simulink model "PMSM_Control_Using_FOC_And_SVPWM"  (R2023b)
settings: Solver=ode23t  StartTime=0.0  StopTime=2.5  MaxStep=1e-4  RelTol=1e-3
undefined symbols (not defined in the file): Acid, Ion, Ld, Lead, Lithium, Lq, sigbuilder_block
libraries: slpidlib x58, spsSeriesRLCBranchLib x40, spsVoltageMeasurementLib x34, spsMosfetLib x24, spsBatteryLib x19, spsPWMGeneratorDCDCLib x17, spsCurrentMeasurementLib x15, spsAlphaBetaZerotodq0Lib x14, spsUniversalBridgeLib x14, spsPermanentMagnetSynchronousMachineLib x14, spsSVPWMGenerator2LevelLib x14, spsabctoAlphaBetaZeroLib x14
(part 3 of 3)

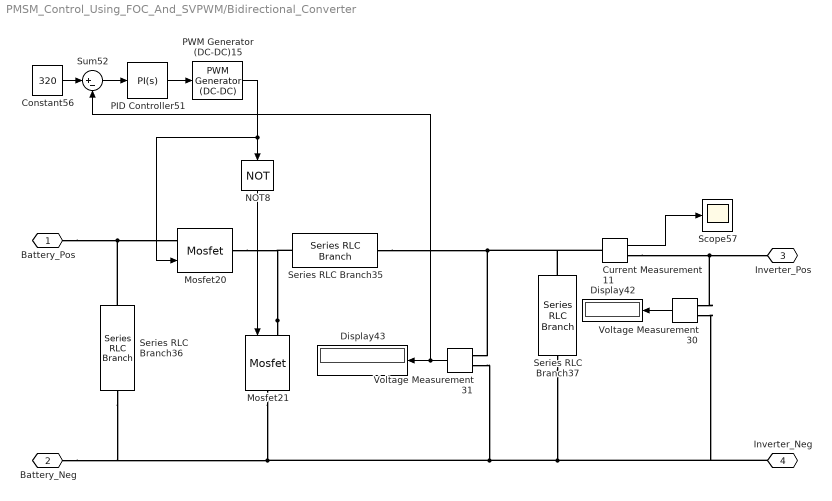
== system PMSM_Control_Using_FOC_And_SVPWM/Bidirectional_Converter ==
  Constant56 : Constant  Value=320
  Current Measurement11 : spsCurrentMeasurementLib/Current Measurement  PhasorSimulation=off  OutputType=Complex  PSBequivalent=0
  Display42 : Display
  Display43 : Display
  Mosfet20 : spsMosfetLib/Mosfet  Ron=0.1  Lon=0  Rd=0.01  Vfd=0  IC=0  Rs=1e5  Cs=inf  Measurements=off
  Mosfet21 : spsMosfetLib/Mosfet  Ron=0.1  Lon=0  Rd=0.01  Vfd=0  IC=0  Rs=1e5  Cs=inf  Measurements=off
  NOT8 : Logic  Operator=NOT  IconShape=distinctive  AllPortsSameDT=off  OutDataTypeStr=boolean
  PID Controller51 : slpidlib/PID Controller  Controller=PI  Form=Parallel  TimeDomain=Continuous-time  UseExternalTs=off  SampleTime=-1  IntegratorMethod=Forward Euler  FilterMethod=Forward Euler  ControllerParametersSource=internal  P=1  I=20  UseKiTs=off  D=0  N=100  UseFilter=on  TunerSelectOption=Transfer Function Based (PID Tuner App)  InitialConditionSource=internal  InitialConditionForIntegrator=0  InitialConditionForFilter=0  DifferentiatorICPrevScaledInput=0  ExternalReset=none  TrackingMode=off  Kt=1  LimitOutput=off  SatLimitsSource=internal  UpperSaturationLimit=inf  LowerSaturationLimit=-inf  LinearizeAsGain=on  AntiWindupMode=none  Kb=1  LimitIntegrator=off  UpperIntegratorSaturationLimit=inf  LowerIntegratorSaturationLimit=-inf  POutMin=[]  POutMax=[]  IOutMin=[]  IOutMax=[]  DOutMin=[]  DOutMax=[]  NOutMin=[]  NOutMax=[]  SumOutMin=[]  SumOutMax=[]  SaturationOutMin=[]  SaturationOutMax=[]  PParamMin=[]  PParamMax=[]  IParamMin=[]  IParamMax=[]  DParamMin=[]  DParamMax=[]  NParamMin=[]  NParamMax=[]  KbParamMin=[]  KbParamMax=[]  KtParamMin=[]  KtParamMax=[]  KbOutMin=[]  KbOutMax=[]  KtOutMin=[]  KtOutMax=[]  IntegratorOutMin=[]  IntegratorOutMax=[]  FilterOutMin=[]  FilterOutMax=[]  SumI1OutMin=[]  SumI1OutMax=[]  SumI2OutMin=[]  SumI2OutMax=[]  SumI3OutMin=[]  SumI3OutMax=[]  SumI4OutMin=[]  SumI4OutMax=[]  SumDOutMin=[]  SumDOutMax=[]  DifferentiatorOutMin=[]  DifferentiatorOutMax=[]  FilterDiffOutCoefMin=[]  FilterDiffOutCoefMax=[]  ReciprocalOutMin=[]  ReciprocalOutMax=[]  SumDenOutMin=[]  SumDenOutMax=[]  SumNumOutMin=[]  SumNumOutMax=[]  DivideOutMin=[]  DivideOutMax=[]  UdiffTsProdOutMin=[]  UdiffTsProdOutMax=[]  NTsProdOutMin=[]  NTsProdOutMax=[]  UintegralTsProdOutMin=[]  UintegralTsProdOutMax=[]  UngainTsProdOutMin=[]  UngainTsProdOutMax=[]  ClampingZeroOutDataTypeStr=Inherit: Inherit via back propagation  ClampingZeroOutMin=[]  ClampingZeroOutMax=[]  FilterDenConstantOutDataTypeStr=Inherit: Inherit via back propagation  FilterDenConstantOutMin=[]  FilterDenConstantOutMax=[]  PCopyOutDataTypeStr=Inherit: Inherit via back propagation  PCopyOutMin=[]  PCopyOutMax=[]  NCopyOutDataTypeStr=Inherit: Inherit via back propagation  NCopyOutMin=[]  NCopyOutMax=[]  IntegratorContinuousStateAttributes=''  IntegratorStateMustResolveToSignalObject=off  IntegratorRTWStateStorageClass=Auto  FilterContinuousStateAttributes=''  FilterStateMustResolveToSignalObject=off  FilterRTWStateStorageClass=Auto  ParallelPVariant=InternalParameters  IdealPVariant=Disabled  IVariant=InternalParameters  DVariant=Disabled  IntegratorVariant=Continuous  SatVariant=Disabled  AWVariant=Passthrough  PCopyVariant=Disabled  TRVariant=Disabled  FdbkBlocksVariant=Forward  IdealPFdbkVariant=Disabled  SatFdbkVariant=Disabled  DerivativeFilterVariant=Disabled  NVariant=Disabled  NCopyVariant=Disabled_SignalSpec  FilterICVariant=Disabled  IntegratorICVariant=InternalICs  ExternalResetVariant=Disabled  TRSumVariant=Passthrough  SumFdbkVariant=Disabled  SumVariant=Sum_PI  TsampFilterVariant=InternalTs  TsampNgainVariant=Passthrough  TsampIntegralVariant=Disabled_SignalSpec  ExternalSaturationOutDataTypeStr=Inherit: Same as second input
  PWM Generator (DC-DC)15 : spsPWMGeneratorDCDCLib/PWM Generator (DC-DC)  Fsw=5000  Ts=0
  Scope57 : Scope
  Series RLC Branch35 : spsSeriesRLCBranchLib/Series RLC Branch  LConnTagsString=__new0  RConnTagsString=__new0  BranchType=L  Resistance=0.0001  Inductance=1e-3  SetiL0=off  InitialCurrent=0  Capacitance=1000e-6  Setx0=off  InitialVoltage=0  Measurements=None
  Series RLC Branch36 : spsSeriesRLCBranchLib/Series RLC Branch  LConnTagsString=__new0  RConnTagsString=__new0  BranchType=RC  Resistance=0.0001  Inductance=1e-3  SetiL0=off  InitialCurrent=0  Capacitance=1000e-6  Setx0=off  InitialVoltage=0  Measurements=None
  Series RLC Branch37 : spsSeriesRLCBranchLib/Series RLC Branch  LConnTagsString=__new0  RConnTagsString=__new0  BranchType=RC  Resistance=0.01  Inductance=1e-3  SetiL0=off  InitialCurrent=0  Capacitance=1e-3  Setx0=off  InitialVoltage=0  Measurements=None
  Sum52 : Sum  Inputs=|+-
  Voltage Measurement30 : spsVoltageMeasurementLib/Voltage Measurement  PhasorSimulation=off  OutputType=Complex  PSBequivalent=0
  Voltage Measurement31 : spsVoltageMeasurementLib/Voltage Measurement  PhasorSimulation=off  OutputType=Complex  PSBequivalent=0
  Battery_Pos : PMIOPort  Side=Left
  Battery_Neg : PMIOPort  Port=2  Side=Left
  Inverter_Pos : PMIOPort  Port=3  Side=Right
  Inverter_Neg : PMIOPort  Port=4  Side=Right
  wires:
  PID Controller51/1 -> PWM Generator (DC-DC)15/1
  Current Measurement11/1 -> Scope57/1
  Constant56/1 -> Sum52/1
  Sum52/1 -> PID Controller51/1
  PWM Generator (DC-DC)15/1 -> Mosfet20/1, NOT8/1
  NOT8/1 -> Mosfet21/1
  Voltage Measurement31/1 -> Sum52/2, Display43/1
  Voltage Measurement30/1 -> Display42/1
  connections:
  Mosfet21/LConn1 -- Series RLC Branch35/LConn1 -- Mosfet20/RConn1
  Series RLC Branch36/LConn1 -- Battery_Pos/RConn1 -- Mosfet20/LConn1
  Current Measurement11/RConn1 -- Voltage Measurement30/LConn1 -- Inverter_Pos/RConn1
  Voltage Measurement31/LConn1 -- Series RLC Branch37/LConn1 -- Current Measurement11/LConn1 -- Series RLC Branch35/RConn1
  Mosfet21/RConn1 -- Voltage Measurement30/LConn2 -- Inverter_Neg/RConn1 -- Series RLC Branch37/RConn1 -- Voltage Measurement31/LConn2 -- Battery_Neg/RConn1 -- Series RLC Branch36/RConn1

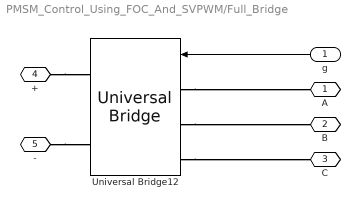
== system PMSM_Control_Using_FOC_And_SVPWM/Full_Bridge ==
  g : Inport
  Universal Bridge12 : spsUniversalBridgeLib/Universal Bridge  Arms=3  SnubberResistance=1e5  SnubberCapacitance=inf  Device=IGBT / Diodes  Ron=1e-3  Lon=0  ForwardVoltages="[  0  0  ]"  ForwardVoltage=0  GTOparameters=[ 10e-6 , 20e-6 ]  IGBTparameters=[ 1e-6 , 2e-6 ]  Measurements=None  Measurements_2=None  converterType=Rectifier
  A : PMIOPort  Side=Left
  B : PMIOPort  Port=2  Side=Left
  C : PMIOPort  Port=3  Side=Left
  + : PMIOPort  Port=4  Side=Right
  - : PMIOPort  Port=5  Side=Right
  wires:
  g/1 -> Universal Bridge12/1
  connections:
  Universal Bridge12/LConn1 -- A/RConn1
  +/RConn1 -- Universal Bridge12/RConn1
  Universal Bridge12/LConn2 -- B/RConn1
  Universal Bridge12/LConn3 -- C/RConn1
  -/RConn1 -- Universal Bridge12/RConn2

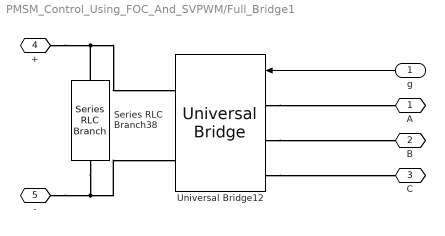
== system PMSM_Control_Using_FOC_And_SVPWM/Full_Bridge1 ==
  g : Inport
  Series RLC Branch38 : spsSeriesRLCBranchLib/Series RLC Branch  LConnTagsString=__new0  RConnTagsString=__new0  BranchType=RC  Resistance=0.01  Inductance=1e-3  SetiL0=off  InitialCurrent=0  Capacitance=1e-3  Setx0=off  InitialVoltage=0  Measurements=None
  Universal Bridge12 : spsUniversalBridgeLib/Universal Bridge  Arms=3  SnubberResistance=1e5  SnubberCapacitance=inf  Device=IGBT / Diodes  Ron=1e-3  Lon=0  ForwardVoltages="[  0  0  ]"  ForwardVoltage=0  GTOparameters=[ 10e-6 , 20e-6 ]  IGBTparameters=[ 1e-6 , 2e-6 ]  Measurements=None  Measurements_2=None  converterType=Rectifier
  A : PMIOPort  Side=Left
  B : PMIOPort  Port=2  Side=Left
  C : PMIOPort  Port=3  Side=Left
  + : PMIOPort  Port=4  Side=Right
  - : PMIOPort  Port=5  Side=Right
  wires:
  g/1 -> Universal Bridge12/1
  connections:
  Universal Bridge12/LConn1 -- A/RConn1
  +/RConn1 -- Series RLC Branch38/LConn1 -- Universal Bridge12/RConn1
  Universal Bridge12/LConn2 -- B/RConn1
  Universal Bridge12/LConn3 -- C/RConn1
  -/RConn1 -- Series RLC Branch38/RConn1 -- Universal Bridge12/RConn2

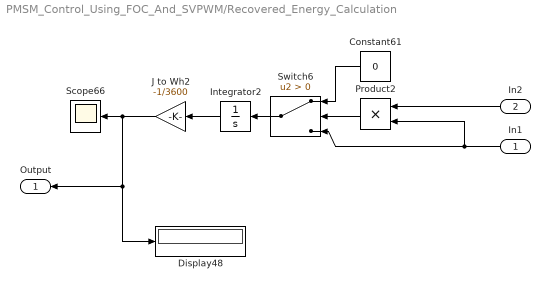
== system PMSM_Control_Using_FOC_And_SVPWM/Recovered_Energy_Calculation ==
  In1 : Inport
  In2 : Inport  Port=2
  Constant61 : Constant  Value=0
  Display48 : Display
  Integrator2 : Integrator
  J to Wh2 : Gain  Gain=-1/3600
  Product2 : Product
  Scope66 : Scope
  Switch6 : Switch  Criteria=u2 > Threshold  SaturateOnIntegerOverflow=off  InputSameDT=off
  Output : Outport
  wires:
  Constant61/1 -> Switch6/1
  Integrator2/1 -> J to Wh2/1
  Switch6/1 -> Integrator2/1
  J to Wh2/1 -> Display48/1, Output/1, Scope66/1
  In2/1 -> Product2/1
  Product2/1 -> Switch6/2
  In1/1 -> Product2/2, Switch6/3

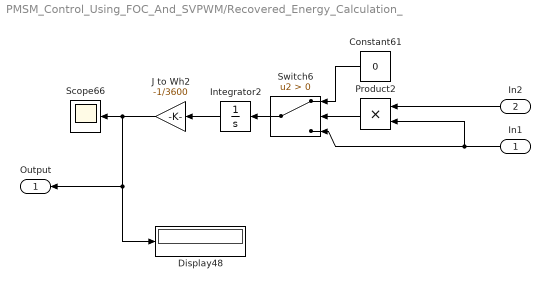
== system PMSM_Control_Using_FOC_And_SVPWM/Recovered_Energy_Calculation_ ==
  In1 : Inport
  In2 : Inport  Port=2
  Constant61 : Constant  Value=0
  Display48 : Display
  Integrator2 : Integrator
  J to Wh2 : Gain  Gain=-1/3600
  Product2 : Product
  Scope66 : Scope
  Switch6 : Switch  Criteria=u2 > Threshold  SaturateOnIntegerOverflow=off  InputSameDT=off
  Output : Outport
  wires:
  Constant61/1 -> Switch6/1
  Integrator2/1 -> J to Wh2/1
  Switch6/1 -> Integrator2/1
  J to Wh2/1 -> Display48/1, Output/1, Scope66/1
  In2/1 -> Product2/1
  Product2/1 -> Switch6/2
  In1/1 -> Product2/2, Switch6/3

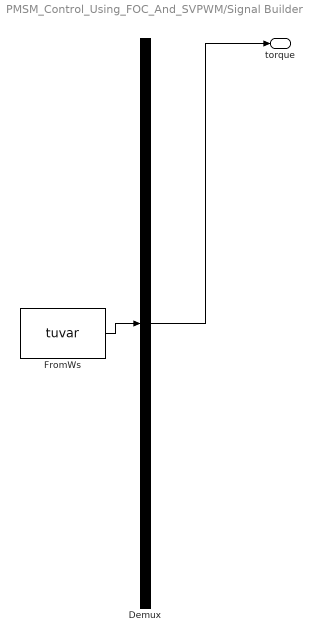
== system PMSM_Control_Using_FOC_And_SVPWM/Signal Builder ==
  Demux : Demux  Tag=STV Demux  Outputs=1
      settings: DisplayOption=none
  FromWs : FromWorkspace  Tag=STV FromWs  VariableName=tuvar
      SigBuilderData=|
      | common.afterFinalStr = 'Extrapolate'
      | common.sampleTime = 0
      | dataSet.timeRange = [0 2.5]
      | dataSet.name = 'Imported_Group 1'
      | sbobj.Name = 'Signal Builder'
      | sbobj.Groups.Name = 'Imported_Group 1'
      | sbobj.Groups.Signals.Name = 'torque'
      | sbobj.Groups.Signals.XData = [0 0.05 0.05 0.5 0.5 0.75 0.75 1.25 1.25 1.65 1.65 2.05 2.05 2.35 2.35 2.5]
      | sbobj.Groups.Signals.YData = [0 0 5 5 4 4 -3 -3 1.5 1.5 5 5 4 4 -1 -1]
      | sbobj.Groups.TimeRange = [0 2.5]
  torque : Outport  VectorParamsAs1DForOutWhenUnconnected=off
  wires:
  Demux/1 -> torque/1
  FromWs/1 -> Demux/1

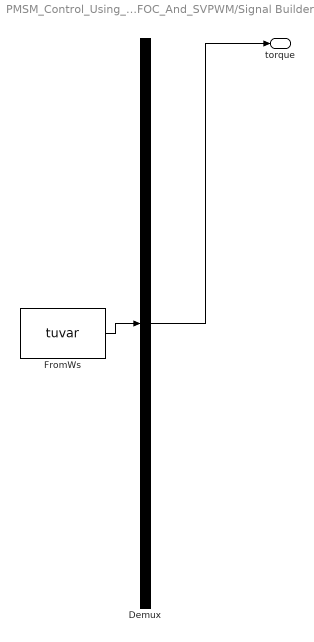
== system PMSM_Control_Using_FOC_And_SVPWM/Signal Builder1 ==
  Demux : Demux  Tag=STV Demux  Outputs=1
      settings: DisplayOption=none
  FromWs : FromWorkspace  Tag=STV FromWs  VariableName=tuvar
      SigBuilderData=|
      | common.afterFinalStr = 'Extrapolate'
      | common.sampleTime = 0
      | dataSet.timeRange = [0 2.5]
      | dataSet.name = 'Imported_Group 1'
      | sbobj.Name = 'Signal Builder'
      | sbobj.Groups.Name = 'Imported_Group 1'
      | sbobj.Groups.Signals.Name = 'torque'
      | sbobj.Groups.Signals.XData = [0 0.05 0.05 0.5 0.5 0.75 0.75 1.25 1.25 1.65 1.65 2.05 2.05 2.35 2.35 2.5]
      | sbobj.Groups.Signals.YData = [0 0 5 5 4 4 -3 -3 1.5 1.5 5 5 4 4 -1 -1]
      | sbobj.Groups.TimeRange = [0 2.5]
  torque : Outport  VectorParamsAs1DForOutWhenUnconnected=off
  wires:
  FromWs/1 -> Demux/1
  Demux/1 -> torque/1

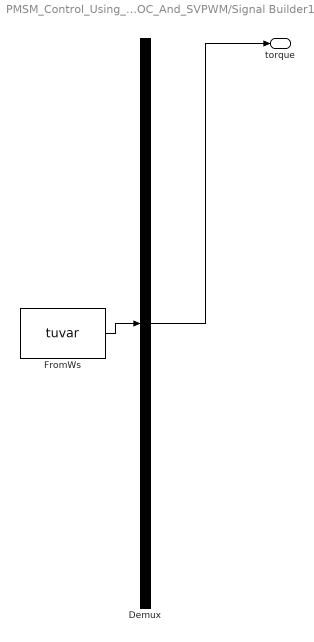
== system PMSM_Control_Using_FOC_And_SVPWM/Signal Builder10 ==
  Demux : Demux  Tag=STV Demux  Outputs=1
      settings: DisplayOption=none
  FromWs : FromWorkspace  Tag=STV FromWs  VariableName=tuvar
      SigBuilderData=|
      | common.afterFinalStr = 'Extrapolate'
      | common.sampleTime = 0
      | dataSet.timeRange = [0 2.5]
      | dataSet.name = 'DownHill_Torque'
      | sbobj.Name = 'Signal Builder'
      | sbobj.Groups.Name = 'DownHill_Torque'
      | sbobj.Groups.Signals.Name = 'torque'
      | sbobj.Groups.Signals.XData = [0 0.05 0.3 0.5 0.8 1.25 1.25 1.65 1.65 2.05 2.35 2.5]
      | sbobj.Groups.Signals.YData = [0 0 -100 -115 -85 -65 -60 -75 -77.5 -50 -40 -1]
      | sbobj.Groups.TimeRange = [0 2.5]
  torque : Outport  VectorParamsAs1DForOutWhenUnconnected=off
  wires:
  FromWs/1 -> Demux/1
  Demux/1 -> torque/1

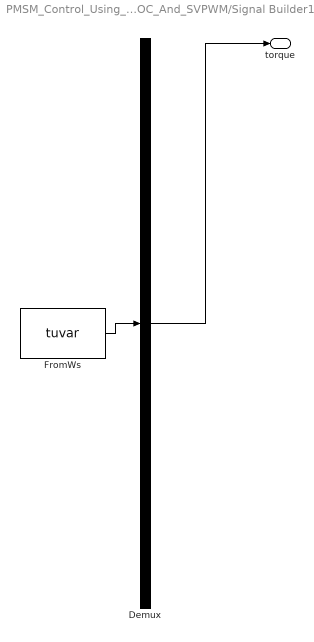
== system PMSM_Control_Using_FOC_And_SVPWM/Signal Builder11 ==
  Demux : Demux  Tag=STV Demux  Outputs=1
      settings: DisplayOption=none
  FromWs : FromWorkspace  Tag=STV FromWs  VariableName=tuvar
      SigBuilderData=|
      | common.afterFinalStr = 'Extrapolate'
      | common.sampleTime = 0
      | dataSet.timeRange = [0 2.5]
      | dataSet.name = 'Flat_Road_Torque'
      | sbobj.Name = 'Signal Builder'
      | sbobj.Groups.Name = 'Flat_Road_Torque'
      | sbobj.Groups.Signals.Name = 'torque'
      | sbobj.Groups.Signals.XData = [0 0.05 0.1 0.3 0.4 0.7 0.8 1.2 1.25 1.6 1.65 2 2.05 2.25 2.35 2.5]
      | sbobj.Groups.Signals.YData = [0 0 8 8 5 5 -8 -8 -3 -3 -7 -7 -8 -8 -1 -1]
      | sbobj.Groups.TimeRange = [0 2.5]
  torque : Outport  VectorParamsAs1DForOutWhenUnconnected=off
  wires:
  FromWs/1 -> Demux/1
  Demux/1 -> torque/1

== system PMSM_Control_Using_FOC_And_SVPWM/Signal Builder13 ==
  Demux : Demux  Tag=STV Demux  Outputs=1
      settings: DisplayOption=none
  FromWs : FromWorkspace  Tag=STV FromWs  VariableName=tuvar
      SigBuilderData=|
      | common.afterFinalStr = 'Extrapolate'
      | common.sampleTime = 0
      | dataSet.timeRange = [0 2.5]
      | dataSet.name = 'Flat_Road_Torque'
      | sbobj.Name = 'Signal Builder'
      | sbobj.Groups.Name = 'Flat_Road_Torque'
      | sbobj.Groups.Signals.Name = 'torque'
      | sbobj.Groups.Signals.XData = [0 0.05 0.1 0.3 0.4 0.7 0.8 1.2 1.25 1.6 1.65 2 2.05 2.25 2.35 2.5]
      | sbobj.Groups.Signals.YData = [0 0 5 5 3 3 -5 -5 -3 -3 -4 -4 -5 -5 -1 -1]
      | sbobj.Groups.TimeRange = [0 2.5]
  torque : Outport  VectorParamsAs1DForOutWhenUnconnected=off
  wires:
  Demux/1 -> torque/1
  FromWs/1 -> Demux/1

== system PMSM_Control_Using_FOC_And_SVPWM/Signal Builder2 ==
  Demux : Demux  Tag=STV Demux  Outputs=1
      settings: DisplayOption=none
  FromWs : FromWorkspace  Tag=STV FromWs  VariableName=tuvar
      SigBuilderData=|
      | common.afterFinalStr = 'Extrapolate'
      | common.sampleTime = 0
      | dataSet.timeRange = [0 2.5]
      | dataSet.name = 'Imported_Group 1'
      | sbobj.Name = 'Signal Builder'
      | sbobj.Groups.Name = 'Imported_Group 1'
      | sbobj.Groups.Signals.Name = 'torque'
      | sbobj.Groups.Signals.XData = [0 0.05 0.05 0.5 0.5 0.75 0.75 1.25 1.25 1.65 1.65 2.05 2.05 2.35 2.35 2.5]
      | sbobj.Groups.Signals.YData = [0 0 5 5 4 4 -3 -3 1.5 1.5 5 5 4 4 -1 -1]
      | sbobj.Groups.TimeRange = [0 2.5]
  torque : Outport  VectorParamsAs1DForOutWhenUnconnected=off
  wires:
  FromWs/1 -> Demux/1
  Demux/1 -> torque/1

== system PMSM_Control_Using_FOC_And_SVPWM/Signal Builder3 ==
  Demux : Demux  Tag=STV Demux  Outputs=1
      settings: DisplayOption=none
  FromWs : FromWorkspace  Tag=STV FromWs  VariableName=tuvar
      SigBuilderData=|
      | common.afterFinalStr = 'Extrapolate'
      | common.sampleTime = 0
      | dataSet.timeRange = [0 2.5]
      | dataSet.name = 'Flat_Road_Torque'
      | sbobj.Name = 'Signal Builder'
      | sbobj.Groups.Name = 'Flat_Road_Torque'
      | sbobj.Groups.Signals.Name = 'torque'
      | sbobj.Groups.Signals.XData = [0 0.05 0.05 0.5 0.5 0.75 0.75 1.25 1.25 1.65 1.65 2.05 2.05 2.35 2.35 2.5]
      | sbobj.Groups.Signals.YData = [0 0 5 5 4 4 -3 -3 1.5 1.5 5 5 4 4 -1 -1]
      | sbobj.Groups.TimeRange = [0 2.5]
  torque : Outport  VectorParamsAs1DForOutWhenUnconnected=off
  wires:
  Demux/1 -> torque/1
  FromWs/1 -> Demux/1

== system PMSM_Control_Using_FOC_And_SVPWM/Signal Builder4 ==
  Demux : Demux  Tag=STV Demux  Outputs=1
      settings: DisplayOption=none
  FromWs : FromWorkspace  Tag=STV FromWs  VariableName=tuvar
      SigBuilderData=|
      | common.afterFinalStr = 'Extrapolate'
      | common.sampleTime = 0
      | dataSet.timeRange = [0 2.5]
      | dataSet.name = 'Imported_Group 1'
      | sbobj.Name = 'Signal Builder'
      | sbobj.Groups.Name = 'Imported_Group 1'
      | sbobj.Groups.Signals.Name = 'torque'
      | sbobj.Groups.Signals.XData = [0 0.05 0.05 0.5 0.5 0.75 0.75 1.25 1.25 1.65 1.65 2.05 2.05 2.35 2.35 2.5]
      | sbobj.Groups.Signals.YData = [0 0 5 5 4 4 -3 -3 1.5 1.5 5 5 4 4 -1 -1]
      | sbobj.Groups.TimeRange = [0 2.5]
  torque : Outport  VectorParamsAs1DForOutWhenUnconnected=off
  wires:
  Demux/1 -> torque/1
  FromWs/1 -> Demux/1

== system PMSM_Control_Using_FOC_And_SVPWM/Signal Builder5 ==
  Demux : Demux  Tag=STV Demux  Outputs=1
      settings: DisplayOption=none
  FromWs : FromWorkspace  Tag=STV FromWs  VariableName=tuvar
      SigBuilderData=|
      | common.afterFinalStr = 'Extrapolate'
      | common.sampleTime = 0
      | dataSet.timeRange = [0 2.5]
      | dataSet.name = 'DownHill_Torque'
      | sbobj.Name = 'Signal Builder'
      | sbobj.Groups.Name = 'DownHill_Torque'
      | sbobj.Groups.Signals.Name = 'torque'
      | sbobj.Groups.Signals.XData = [0 0.05 0.3 0.5 0.8 1.25 1.25 1.65 1.65 2.05 2.35 2.5]
      | sbobj.Groups.Signals.YData = [0 0 -100 -115 -85 -65 -60 -75 -77.5 -50 -40 -1]
      | sbobj.Groups.TimeRange = [0 2.5]
  torque : Outport  VectorParamsAs1DForOutWhenUnconnected=off
  wires:
  Demux/1 -> torque/1
  FromWs/1 -> Demux/1

== system PMSM_Control_Using_FOC_And_SVPWM/Signal Builder6 ==
  Demux : Demux  Tag=STV Demux  Outputs=1
      settings: DisplayOption=none
  FromWs : FromWorkspace  Tag=STV FromWs  VariableName=tuvar
      SigBuilderData=|
      | common.afterFinalStr = 'Extrapolate'
      | common.sampleTime = 0
      | dataSet.timeRange = [0 2.5]
      | dataSet.name = 'Flat_Road_Torque'
      | sbobj.Name = 'Signal Builder'
      | sbobj.Groups.Name = 'Flat_Road_Torque'
      | sbobj.Groups.Signals.Name = 'torque'
      | sbobj.Groups.Signals.XData = [0 0.05 0.05 0.5 0.5 0.75 0.75 1.25 1.25 1.65 1.65 2.05 2.05 2.35 2.35 2.5]
      | sbobj.Groups.Signals.YData = [0 0 5 5 4 4 -3 -3 1.5 1.5 5 5 4 4 -1 -1]
      | sbobj.Groups.TimeRange = [0 2.5]
  torque : Outport  VectorParamsAs1DForOutWhenUnconnected=off
  wires:
  FromWs/1 -> Demux/1
  Demux/1 -> torque/1

== system PMSM_Control_Using_FOC_And_SVPWM/Signal Builder7 ==
  Demux : Demux  Tag=STV Demux  Outputs=1
      settings: DisplayOption=none
  FromWs : FromWorkspace  Tag=STV FromWs  VariableName=tuvar
      SigBuilderData=|
      | common.afterFinalStr = 'Extrapolate'
      | common.sampleTime = 0
      | dataSet.timeRange = [0 2.5]
      | dataSet.name = 'Flat_Road_Torque'
      | sbobj.Name = 'Signal Builder'
      | sbobj.Groups.Name = 'Flat_Road_Torque'
      | sbobj.Groups.Signals.Name = 'torque'
      | sbobj.Groups.Signals.XData = [0 0.05 0.05 0.5 0.5 0.75 0.75 1.25 1.25 1.65 1.65 2.05 2.05 2.35 2.35 2.5]
      | sbobj.Groups.Signals.YData = [0 0 5 5 4 4 -3 -3 1.5 1.5 5 5 4 4 -1 -1]
      | sbobj.Groups.TimeRange = [0 2.5]
  torque : Outport  VectorParamsAs1DForOutWhenUnconnected=off
  wires:
  Demux/1 -> torque/1
  FromWs/1 -> Demux/1

== system PMSM_Control_Using_FOC_And_SVPWM/Signal Builder8 ==
  Demux : Demux  Tag=STV Demux  Outputs=1
      settings: DisplayOption=none
  FromWs : FromWorkspace  Tag=STV FromWs  VariableName=tuvar
      SigBuilderData=|
      | common.afterFinalStr = 'Extrapolate'
      | common.sampleTime = 0
      | dataSet.timeRange = [0 2.5]
      | dataSet.name = 'DownHill_Torque'
      | sbobj.Name = 'Signal Builder'
      | sbobj.Groups.Name = 'DownHill_Torque'
      | sbobj.Groups.Signals.Name = 'torque'
      | sbobj.Groups.Signals.XData = [0 0.05 0.3 0.5 0.8 1.25 1.25 1.65 1.65 2.05 2.35 2.5]
      | sbobj.Groups.Signals.YData = [0 0 -100 -115 -85 -65 -60 -75 -77.5 -50 -40 -1]
      | sbobj.Groups.TimeRange = [0 2.5]
  torque : Outport  VectorParamsAs1DForOutWhenUnconnected=off
  wires:
  Demux/1 -> torque/1
  FromWs/1 -> Demux/1

== system PMSM_Control_Using_FOC_And_SVPWM/Signal Builder9 ==
  Demux : Demux  Tag=STV Demux  Outputs=1
      settings: DisplayOption=none
  FromWs : FromWorkspace  Tag=STV FromWs  VariableName=tuvar
      SigBuilderData=|
      | common.afterFinalStr = 'Extrapolate'
      | common.sampleTime = 0
      | dataSet.timeRange = [0 2.5]
      | dataSet.name = 'UpHill_Torque'
      | sbobj.Name = 'Signal Builder'
      | sbobj.Groups.Name = 'UpHill_Torque'
      | sbobj.Groups.Signals.Name = 'torque'
      | sbobj.Groups.Signals.XData = [0 0.05 0.05 0.2 0.2 0.25 0.25 1.25 1.25 1.65 1.65 2.05 2.05 2.35 2.35 2.5]
      | sbobj.Groups.Signals.YData = [0 0 5 5 4 4 -3 -3 -4.5 -4.5 -5 -5 -4 -4 -1 -1]
      | sbobj.Groups.TimeRange = [0 2.5]
  torque : Outport  VectorParamsAs1DForOutWhenUnconnected=off
  wires:
  Demux/1 -> torque/1
  FromWs/1 -> Demux/1

== system PMSM_Control_Using_FOC_And_SVPWM/Speed_Path ==
  Demux : Demux  Tag=STV Demux  Outputs=1
      settings: DisplayOption=none
  FromWs : FromWorkspace  Tag=STV FromWs  VariableName=tuvar
      SigBuilderData=|
      | common.afterFinalStr = 'Extrapolate'
      | common.sampleTime = 0
      | dataSet.timeRange = [0 2.5]
      | dataSet.name = 'Imported_Group 1'
      | sbobj.Name = 'Signal Builder'
      | sbobj.Groups.Name = 'Imported_Group 1'
      | sbobj.Groups.Signals.Name = 'speed'
      | sbobj.Groups.Signals.XData = [0 0 0.5 0.75 1.25 1.65 2.05 2.35 2.5]
      | sbobj.Groups.Signals.YData = [0 0 2500 2500 1000 1000 2000 2000 1000]
      | sbobj.Groups.TimeRange = [0 2.5]
  speed : Outport  VectorParamsAs1DForOutWhenUnconnected=off
  wires:
  Demux/1 -> speed/1
  FromWs/1 -> Demux/1

== system PMSM_Control_Using_FOC_And_SVPWM/Speed_Path1 ==
  Demux : Demux  Tag=STV Demux  Outputs=1
      settings: DisplayOption=none
  FromWs : FromWorkspace  Tag=STV FromWs  VariableName=tuvar
      SigBuilderData=|
      | common.afterFinalStr = 'Extrapolate'
      | common.sampleTime = 0
      | dataSet.timeRange = [0 2.5]
      | dataSet.name = 'Imported_Group 1'
      | sbobj.Name = 'Signal Builder'
      | sbobj.Groups.Name = 'Imported_Group 1'
      | sbobj.Groups.Signals.Name = 'speed'
      | sbobj.Groups.Signals.XData = [0 0 0.5 0.75 1.25 1.65 2.05 2.35 2.5]
      | sbobj.Groups.Signals.YData = [0 0 2500 2500 1000 1000 2000 2000 1000]
      | sbobj.Groups.TimeRange = [0 2.5]
  speed : Outport  VectorParamsAs1DForOutWhenUnconnected=off
  wires:
  FromWs/1 -> Demux/1
  Demux/1 -> speed/1

== system PMSM_Control_Using_FOC_And_SVPWM/Speed_Path10 ==
  Demux : Demux  Tag=STV Demux  Outputs=1
      settings: DisplayOption=none
  FromWs : FromWorkspace  Tag=STV FromWs  VariableName=tuvar
      SigBuilderData=|
      | common.afterFinalStr = 'Extrapolate'
      | common.sampleTime = 0
      | dataSet.timeRange = [0 2.5]
      | dataSet.name = 'DownHill_Speed'
      | sbobj.Name = 'Signal Builder'
      | sbobj.Groups.Name = 'DownHill_Speed'
      | sbobj.Groups.Signals.Name = 'speed'
      | sbobj.Groups.Signals.XData = [0 0.5 0.75 1.25 1.65 2.05 2.35 2.5]
      | sbobj.Groups.Signals.YData = [0 450 500 350 600 500 300 100]
      | sbobj.Groups.TimeRange = [0 2.5]
  speed : Outport  VectorParamsAs1DForOutWhenUnconnected=off
  wires:
  FromWs/1 -> Demux/1
  Demux/1 -> speed/1

== system PMSM_Control_Using_FOC_And_SVPWM/Speed_Path12 ==
  Demux : Demux  Tag=STV Demux  Outputs=1
      settings: DisplayOption=none
  FromWs : FromWorkspace  Tag=STV FromWs  VariableName=tuvar
      SigBuilderData=|
      | common.afterFinalStr = 'Extrapolate'
      | common.sampleTime = 0
      | dataSet(1).timeRange = [0 2.5]
      | dataSet(1).name = 'Flat_Road_Speed'
      | dataSet(2).timeRange = [0 2.5]
      | dataSet(2).name = 'Flat_Road_Speed1'
      | sbobj.Name = 'Signal Builder'
      | sbobj.Groups(1).Name = 'Flat_Road_Speed'
      | sbobj.Groups(1).Signals.Name = 'speed'
      | sbobj.Groups(1).Signals.XData = [0 0.5 0.75 1 1.3 1.5 2 2.5]
      | sbobj.Groups(1).Signals.YData = [0 1800 1800 1000 1000 1500 1500 0]
      | sbobj.Groups(1).TimeRange = [0 2.5]
      | sbobj.Groups(2).Name = 'Flat_Road_Speed1'
      | sbobj.Groups(2).Signals.Name = 'speed'
      | sbobj.Groups(2).Signals.XData = [0 0.5 0.75 1.25 1.65 2.05 2.35 2.5]
      | sbobj.Groups(2).Signals.YData = [0 2500 2500 1000 1000 2000 2000 1000]
      | sbobj.Groups(2).TimeRange = [0 2.5]
  speed : Outport  VectorParamsAs1DForOutWhenUnconnected=off
  wires:
  Demux/1 -> speed/1
  FromWs/1 -> Demux/1

== system PMSM_Control_Using_FOC_And_SVPWM/Speed_Path2 ==
  Demux : Demux  Tag=STV Demux  Outputs=1
      settings: DisplayOption=none
  FromWs : FromWorkspace  Tag=STV FromWs  VariableName=tuvar
      SigBuilderData=|
      | common.afterFinalStr = 'Extrapolate'
      | common.sampleTime = 0
      | dataSet.timeRange = [0 2.5]
      | dataSet.name = 'Imported_Group 1'
      | sbobj.Name = 'Signal Builder'
      | sbobj.Groups.Name = 'Imported_Group 1'
      | sbobj.Groups.Signals.Name = 'speed'
      | sbobj.Groups.Signals.XData = [0 0.5 0.75 1.25 1.65 2.05 2.35 2.5]
      | sbobj.Groups.Signals.YData = [0 2500 2500 1000 1000 2000 2000 1000]
      | sbobj.Groups.TimeRange = [0 2.5]
  speed : Outport  VectorParamsAs1DForOutWhenUnconnected=off
  wires:
  FromWs/1 -> Demux/1
  Demux/1 -> speed/1

== system PMSM_Control_Using_FOC_And_SVPWM/Speed_Path3 ==
  Demux : Demux  Tag=STV Demux  Outputs=1
      settings: DisplayOption=none
  FromWs : FromWorkspace  Tag=STV FromWs  VariableName=tuvar
      SigBuilderData=|
      | common.afterFinalStr = 'Extrapolate'
      | common.sampleTime = 0
      | dataSet(1).timeRange = [0 2.5]
      | dataSet(1).name = 'Flat_Road_Speed'
      | dataSet(2).timeRange = [0 2.5]
      | dataSet(2).name = 'Flat_Road_Speed1'
      | sbobj.Name = 'Signal Builder'
      | sbobj.Groups(1).Name = 'Flat_Road_Speed'
      | sbobj.Groups(1).Signals.Name = 'speed'
      | sbobj.Groups(1).Signals.XData = [0 0.5 0.75 1 1.5 1.8 2.2 2.5]
      | sbobj.Groups(1).Signals.YData = [0 1200 1200 600 600 1000 1000 200]
      | sbobj.Groups(1).TimeRange = [0 2.5]
      | sbobj.Groups(2).Name = 'Flat_Road_Speed1'
      | sbobj.Groups(2).Signals.Name = 'speed'
      | sbobj.Groups(2).Signals.XData = [0 0.5 0.75 1.25 1.65 2.05 2.35 2.5]
      | sbobj.Groups(2).Signals.YData = [0 2500 2500 1000 1000 2000 2000 1000]
      | sbobj.Groups(2).TimeRange = [0 2.5]
  speed : Outport  VectorParamsAs1DForOutWhenUnconnected=off
  wires:
  FromWs/1 -> Demux/1
  Demux/1 -> speed/1

== system PMSM_Control_Using_FOC_And_SVPWM/Speed_Path4 ==
  Demux : Demux  Tag=STV Demux  Outputs=1
      settings: DisplayOption=none
  FromWs : FromWorkspace  Tag=STV FromWs  VariableName=tuvar
      SigBuilderData=|
      | common.afterFinalStr = 'Extrapolate'
      | common.sampleTime = 0
      | dataSet.timeRange = [0 2.5]
      | dataSet.name = 'Imported_Group 1'
      | sbobj.Name = 'Signal Builder'
      | sbobj.Groups.Name = 'Imported_Group 1'
      | sbobj.Groups.Signals.Name = 'speed'
      | sbobj.Groups.Signals.XData = [0 0.5 0.75 1.25 1.65 2.05 2.35 2.5]
      | sbobj.Groups.Signals.YData = [0 2500 2500 1000 1000 2000 2000 1000]
      | sbobj.Groups.TimeRange = [0 2.5]
  speed : Outport  VectorParamsAs1DForOutWhenUnconnected=off
  wires:
  Demux/1 -> speed/1
  FromWs/1 -> Demux/1

== system PMSM_Control_Using_FOC_And_SVPWM/Speed_Path5 ==
  Demux : Demux  Tag=STV Demux  Outputs=1
      settings: DisplayOption=none
  FromWs : FromWorkspace  Tag=STV FromWs  VariableName=tuvar
      SigBuilderData=|
      | common.afterFinalStr = 'Extrapolate'
      | common.sampleTime = 0
      | dataSet.timeRange = [0 2.5]
      | dataSet.name = 'DownHill_Speed'
      | sbobj.Name = 'Signal Builder'
      | sbobj.Groups.Name = 'DownHill_Speed'
      | sbobj.Groups.Signals.Name = 'speed'
      | sbobj.Groups.Signals.XData = [0 0.5 0.75 1.25 1.65 2.05 2.35 2.5]
      | sbobj.Groups.Signals.YData = [0 450 500 350 600 500 300 100]
      | sbobj.Groups.TimeRange = [0 2.5]
  speed : Outport  VectorParamsAs1DForOutWhenUnconnected=off
  wires:
  Demux/1 -> speed/1
  FromWs/1 -> Demux/1

== system PMSM_Control_Using_FOC_And_SVPWM/Speed_Path6 ==
  Demux : Demux  Tag=STV Demux  Outputs=1
      settings: DisplayOption=none
  FromWs : FromWorkspace  Tag=STV FromWs  VariableName=tuvar
      SigBuilderData=|
      | common.afterFinalStr = 'Extrapolate'
      | common.sampleTime = 0
      | dataSet(1).timeRange = [0 2.5]
      | dataSet(1).name = 'Flat_Road_Speed'
      | dataSet(2).timeRange = [0 2.5]
      | dataSet(2).name = 'Flat_Road_Speed1'
      | sbobj.Name = 'Signal Builder'
      | sbobj.Groups(1).Name = 'Flat_Road_Speed'
      | sbobj.Groups(1).Signals.Name = 'speed'
      | sbobj.Groups(1).Signals.XData = [0 0.5 0.75 1 1.5 1.8 2.2 2.5]
      | sbobj.Groups(1).Signals.YData = [0 1200 1200 600 600 1000 1000 200]
      | sbobj.Groups(1).TimeRange = [0 2.5]
      | sbobj.Groups(2).Name = 'Flat_Road_Speed1'
      | sbobj.Groups(2).Signals.Name = 'speed'
      | sbobj.Groups(2).Signals.XData = [0 0.5 0.75 1.25 1.65 2.05 2.35 2.5]
      | sbobj.Groups(2).Signals.YData = [0 2500 2500 1000 1000 2000 2000 1000]
      | sbobj.Groups(2).TimeRange = [0 2.5]
  speed : Outport  VectorParamsAs1DForOutWhenUnconnected=off
  wires:
  FromWs/1 -> Demux/1
  Demux/1 -> speed/1

== system PMSM_Control_Using_FOC_And_SVPWM/Speed_Path7 ==
  Demux : Demux  Tag=STV Demux  Outputs=1
      settings: DisplayOption=none
  FromWs : FromWorkspace  Tag=STV FromWs  VariableName=tuvar
      SigBuilderData=|
      | common.afterFinalStr = 'Extrapolate'
      | common.sampleTime = 0
      | dataSet(1).timeRange = [0 2.5]
      | dataSet(1).name = 'Flat_Road_Speed'
      | dataSet(2).timeRange = [0 2.5]
      | dataSet(2).name = 'Flat_Road_Speed1'
      | sbobj.Name = 'Signal Builder'
      | sbobj.Groups(1).Name = 'Flat_Road_Speed'
      | sbobj.Groups(1).Signals.Name = 'speed'
      | sbobj.Groups(1).Signals.XData = [0 0.5 0.75 1 1.5 1.8 2.2 2.5]
      | sbobj.Groups(1).Signals.YData = [0 1200 1200 600 600 1000 1000 200]
      | sbobj.Groups(1).TimeRange = [0 2.5]
      | sbobj.Groups(2).Name = 'Flat_Road_Speed1'
      | sbobj.Groups(2).Signals.Name = 'speed'
      | sbobj.Groups(2).Signals.XData = [0 0.5 0.75 1.25 1.65 2.05 2.35 2.5]
      | sbobj.Groups(2).Signals.YData = [0 2500 2500 1000 1000 2000 2000 1000]
      | sbobj.Groups(2).TimeRange = [0 2.5]
  speed : Outport  VectorParamsAs1DForOutWhenUnconnected=off
  wires:
  Demux/1 -> speed/1
  FromWs/1 -> Demux/1

== system PMSM_Control_Using_FOC_And_SVPWM/Speed_Path8 ==
  Demux : Demux  Tag=STV Demux  Outputs=1
      settings: DisplayOption=none
  FromWs : FromWorkspace  Tag=STV FromWs  VariableName=tuvar
      SigBuilderData=|
      | common.afterFinalStr = 'Extrapolate'
      | common.sampleTime = 0
      | dataSet.timeRange = [0 2.5]
      | dataSet.name = 'DownHill_Speed'
      | sbobj.Name = 'Signal Builder'
      | sbobj.Groups.Name = 'DownHill_Speed'
      | sbobj.Groups.Signals.Name = 'speed'
      | sbobj.Groups.Signals.XData = [0 0.5 0.75 1.25 1.65 2.05 2.35 2.5]
      | sbobj.Groups.Signals.YData = [0 450 500 350 600 500 300 100]
      | sbobj.Groups.TimeRange = [0 2.5]
  speed : Outport  VectorParamsAs1DForOutWhenUnconnected=off
  wires:
  Demux/1 -> speed/1
  FromWs/1 -> Demux/1

== system PMSM_Control_Using_FOC_And_SVPWM/Speed_Path9 ==
  Demux : Demux  Tag=STV Demux  Outputs=1
      settings: DisplayOption=none
  FromWs : FromWorkspace  Tag=STV FromWs  VariableName=tuvar
      SigBuilderData=|
      | common.afterFinalStr = 'Extrapolate'
      | common.sampleTime = 0
      | dataSet.timeRange = [0 2.5]
      | dataSet.name = 'UpHill_Speed'
      | sbobj.Name = 'Signal Builder'
      | sbobj.Groups.Name = 'UpHill_Speed'
      | sbobj.Groups.Signals.Name = 'speed'
      | sbobj.Groups.Signals.XData = [0 0.5 0.75 1.25 1.65 2.05 2.35 2.5]
      | sbobj.Groups.Signals.YData = [0 2500 2500 1400 1400 800 600 100]
      | sbobj.Groups.TimeRange = [0 2.5]
  speed : Outport  VectorParamsAs1DForOutWhenUnconnected=off
  wires:
  Demux/1 -> speed/1
  FromWs/1 -> Demux/1

== system PMSM_Control_Using_FOC_And_SVPWM/Speed_Ref ==
  Demux : Demux  Tag=STV Demux  Outputs=1
      settings: DisplayOption=none
  FromWs : FromWorkspace  Tag=STV FromWs  VariableName=tuvar
      SigBuilderData=|
      | common.afterFinalStr = 'Extrapolate'
      | common.sampleTime = 0
      | dataSet(1).timeRange = [0 2.5]
      | dataSet(1).name = 'Flat_Road_Speed'
      | dataSet(2).timeRange = [0 2.5]
      | dataSet(2).name = 'Flat_Road_Speed1'
      | sbobj.Name = 'Signal Builder'
      | sbobj.Groups(1).Name = 'Flat_Road_Speed'
      | sbobj.Groups(1).Signals.Name = 'speed'
      | sbobj.Groups(1).Signals.XData = [0 0.5 0.75 1 1.3 1.5 2 2.5]
      | sbobj.Groups(1).Signals.YData = [0 1800 1800 1000 1000 1500 1500 0]
      | sbobj.Groups(1).TimeRange = [0 2.5]
      | sbobj.Groups(2).Name = 'Flat_Road_Speed1'
      | sbobj.Groups(2).Signals.Name = 'speed'
      | sbobj.Groups(2).Signals.XData = [0 0.5 0.75 1.25 1.65 2.05 2.35 2.5]
      | sbobj.Groups(2).Signals.YData = [0 2500 2500 1000 1000 2000 2000 1000]
      | sbobj.Groups(2).TimeRange = [0 2.5]
  speed : Outport  VectorParamsAs1DForOutWhenUnconnected=off
  wires:
  FromWs/1 -> Demux/1
  Demux/1 -> speed/1

== system PMSM_Control_Using_FOC_And_SVPWM/Speed_Ref1 ==
  Demux : Demux  Tag=STV Demux  Outputs=1
      settings: DisplayOption=none
  FromWs : FromWorkspace  Tag=STV FromWs  VariableName=tuvar
      SigBuilderData=|
      | common.afterFinalStr = 'Extrapolate'
      | common.sampleTime = 0
      | dataSet(1).timeRange = [0 2.5]
      | dataSet(1).name = 'Flat_Road_Speed'
      | dataSet(2).timeRange = [0 2.5]
      | dataSet(2).name = 'Flat_Road_Speed1'
      | sbobj.Name = 'Signal Builder'
      | sbobj.Groups(1).Name = 'Flat_Road_Speed'
      | sbobj.Groups(1).Signals.Name = 'speed'
      | sbobj.Groups(1).Signals.XData = [0 0.5 0.75 1 1.3 1.5 2 2.5]
      | sbobj.Groups(1).Signals.YData = [0 1800 1800 1000 1000 1500 1500 0]
      | sbobj.Groups(1).TimeRange = [0 2.5]
      | sbobj.Groups(2).Name = 'Flat_Road_Speed1'
      | sbobj.Groups(2).Signals.Name = 'speed'
      | sbobj.Groups(2).Signals.XData = [0 0.5 0.75 1.25 1.65 2.05 2.35 2.5]
      | sbobj.Groups(2).Signals.YData = [0 2500 2500 1000 1000 2000 2000 1000]
      | sbobj.Groups(2).TimeRange = [0 2.5]
  speed : Outport  VectorParamsAs1DForOutWhenUnconnected=off
  wires:
  FromWs/1 -> Demux/1
  Demux/1 -> speed/1

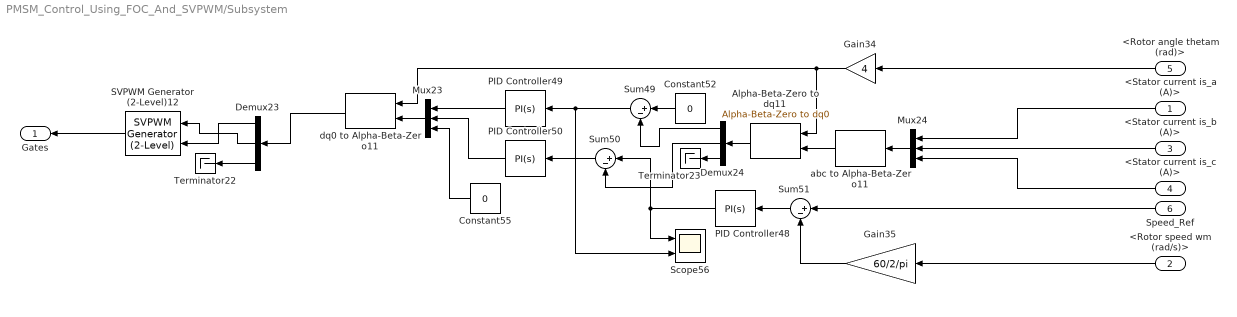
== system PMSM_Control_Using_FOC_And_SVPWM/Subsystem ==
  <Stator current is_a (A)> : Inport
  <Rotor speed wm (rad/s)> : Inport  Port=2
  <Stator current is_b (A)> : Inport  Port=3
  <Stator current is_c (A)> : Inport  Port=4
  <Rotor angle thetam (rad)> : Inport  Port=5
  Speed_Ref : Inport  Port=6
  Alpha-Beta-Zero to dq11 : spsAlphaBetaZerotodq0Lib/Alpha-Beta-Zero to dq0  Alignment=90 degrees behind phase A axis
  Constant52 : Constant  Value=0
  Constant55 : Constant  Value=0
  Demux23 : Demux  Outputs=3
  Demux24 : Demux  Outputs=3
  Gain34 : Gain  Gain=4
  Gain35 : Gain  Gain=60/2/pi
  Mux23 : Mux  Inputs=3
  Mux24 : Mux  Inputs=3
  PID Controller48 : slpidlib/PID Controller  Controller=PI  Form=Parallel  TimeDomain=Continuous-time  UseExternalTs=off  SampleTime=-1  IntegratorMethod=Forward Euler  FilterMethod=Forward Euler  ControllerParametersSource=internal  P=0.5  I=10  UseKiTs=off  D=0  N=100  UseFilter=on  TunerSelectOption=Transfer Function Based (PID Tuner App)  InitialConditionSource=internal  InitialConditionForIntegrator=0  InitialConditionForFilter=0  DifferentiatorICPrevScaledInput=0  ExternalReset=none  TrackingMode=off  Kt=1  LimitOutput=off  SatLimitsSource=internal  UpperSaturationLimit=inf  LowerSaturationLimit=-inf  LinearizeAsGain=on  AntiWindupMode=none  Kb=1  LimitIntegrator=off  UpperIntegratorSaturationLimit=inf  LowerIntegratorSaturationLimit=-inf  POutMin=[]  POutMax=[]  IOutMin=[]  IOutMax=[]  DOutMin=[]  DOutMax=[]  NOutMin=[]  NOutMax=[]  SumOutMin=[]  SumOutMax=[]  SaturationOutMin=[]  SaturationOutMax=[]  PParamMin=[]  PParamMax=[]  IParamMin=[]  IParamMax=[]  DParamMin=[]  DParamMax=[]  NParamMin=[]  NParamMax=[]  KbParamMin=[]  KbParamMax=[]  KtParamMin=[]  KtParamMax=[]  KbOutMin=[]  KbOutMax=[]  KtOutMin=[]  KtOutMax=[]  IntegratorOutMin=[]  IntegratorOutMax=[]  FilterOutMin=[]  FilterOutMax=[]  SumI1OutMin=[]  SumI1OutMax=[]  SumI2OutMin=[]  SumI2OutMax=[]  SumI3OutMin=[]  SumI3OutMax=[]  SumI4OutMin=[]  SumI4OutMax=[]  SumDOutMin=[]  SumDOutMax=[]  DifferentiatorOutMin=[]  DifferentiatorOutMax=[]  FilterDiffOutCoefMin=[]  FilterDiffOutCoefMax=[]  ReciprocalOutMin=[]  ReciprocalOutMax=[]  SumDenOutMin=[]  SumDenOutMax=[]  SumNumOutMin=[]  SumNumOutMax=[]  DivideOutMin=[]  DivideOutMax=[]  UdiffTsProdOutMin=[]  UdiffTsProdOutMax=[]  NTsProdOutMin=[]  NTsProdOutMax=[]  UintegralTsProdOutMin=[]  UintegralTsProdOutMax=[]  UngainTsProdOutMin=[]  UngainTsProdOutMax=[]  ClampingZeroOutDataTypeStr=Inherit: Inherit via back propagation  ClampingZeroOutMin=[]  ClampingZeroOutMax=[]  FilterDenConstantOutDataTypeStr=Inherit: Inherit via back propagation  FilterDenConstantOutMin=[]  FilterDenConstantOutMax=[]  PCopyOutDataTypeStr=Inherit: Inherit via back propagation  PCopyOutMin=[]  PCopyOutMax=[]  NCopyOutDataTypeStr=Inherit: Inherit via back propagation  NCopyOutMin=[]  NCopyOutMax=[]  IntegratorContinuousStateAttributes=''  IntegratorStateMustResolveToSignalObject=off  IntegratorRTWStateStorageClass=Auto  FilterContinuousStateAttributes=''  FilterStateMustResolveToSignalObject=off  FilterRTWStateStorageClass=Auto  ParallelPVariant=InternalParameters  IdealPVariant=Disabled  IVariant=InternalParameters  DVariant=Disabled  IntegratorVariant=Continuous  SatVariant=Disabled  AWVariant=Passthrough  PCopyVariant=Disabled  TRVariant=Disabled  FdbkBlocksVariant=Forward  IdealPFdbkVariant=Disabled  SatFdbkVariant=Disabled  DerivativeFilterVariant=Disabled  NVariant=Disabled  NCopyVariant=Disabled_SignalSpec  FilterICVariant=Disabled  IntegratorICVariant=InternalICs  ExternalResetVariant=Disabled  TRSumVariant=Passthrough  SumFdbkVariant=Disabled  SumVariant=Sum_PI  TsampFilterVariant=InternalTs  TsampNgainVariant=Passthrough  TsampIntegralVariant=Disabled_SignalSpec  ExternalSaturationOutDataTypeStr=Inherit: Same as second input
  PID Controller49 : slpidlib/PID Controller  Controller=PI  Form=Parallel  TimeDomain=Continuous-time  UseExternalTs=off  SampleTime=-1  IntegratorMethod=Forward Euler  FilterMethod=Forward Euler  ControllerParametersSource=internal  P=10  I=2000  UseKiTs=off  D=0  N=100  UseFilter=on  TunerSelectOption=Transfer Function Based (PID Tuner App)  InitialConditionSource=internal  InitialConditionForIntegrator=0  InitialConditionForFilter=0  DifferentiatorICPrevScaledInput=0  ExternalReset=none  TrackingMode=off  Kt=1  LimitOutput=off  SatLimitsSource=internal  UpperSaturationLimit=inf  LowerSaturationLimit=-inf  LinearizeAsGain=on  AntiWindupMode=none  Kb=1  LimitIntegrator=off  UpperIntegratorSaturationLimit=inf  LowerIntegratorSaturationLimit=-inf  POutMin=[]  POutMax=[]  IOutMin=[]  IOutMax=[]  DOutMin=[]  DOutMax=[]  NOutMin=[]  NOutMax=[]  SumOutMin=[]  SumOutMax=[]  SaturationOutMin=[]  SaturationOutMax=[]  PParamMin=[]  PParamMax=[]  IParamMin=[]  IParamMax=[]  DParamMin=[]  DParamMax=[]  NParamMin=[]  NParamMax=[]  KbParamMin=[]  KbParamMax=[]  KtParamMin=[]  KtParamMax=[]  KbOutMin=[]  KbOutMax=[]  KtOutMin=[]  KtOutMax=[]  IntegratorOutMin=[]  IntegratorOutMax=[]  FilterOutMin=[]  FilterOutMax=[]  SumI1OutMin=[]  SumI1OutMax=[]  SumI2OutMin=[]  SumI2OutMax=[]  SumI3OutMin=[]  SumI3OutMax=[]  SumI4OutMin=[]  SumI4OutMax=[]  SumDOutMin=[]  SumDOutMax=[]  DifferentiatorOutMin=[]  DifferentiatorOutMax=[]  FilterDiffOutCoefMin=[]  FilterDiffOutCoefMax=[]  ReciprocalOutMin=[]  ReciprocalOutMax=[]  SumDenOutMin=[]  SumDenOutMax=[]  SumNumOutMin=[]  SumNumOutMax=[]  DivideOutMin=[]  DivideOutMax=[]  UdiffTsProdOutMin=[]  UdiffTsProdOutMax=[]  NTsProdOutMin=[]  NTsProdOutMax=[]  UintegralTsProdOutMin=[]  UintegralTsProdOutMax=[]  UngainTsProdOutMin=[]  UngainTsProdOutMax=[]  ClampingZeroOutDataTypeStr=Inherit: Inherit via back propagation  ClampingZeroOutMin=[]  ClampingZeroOutMax=[]  FilterDenConstantOutDataTypeStr=Inherit: Inherit via back propagation  FilterDenConstantOutMin=[]  FilterDenConstantOutMax=[]  PCopyOutDataTypeStr=Inherit: Inherit via back propagation  PCopyOutMin=[]  PCopyOutMax=[]  NCopyOutDataTypeStr=Inherit: Inherit via back propagation  NCopyOutMin=[]  NCopyOutMax=[]  IntegratorContinuousStateAttributes=''  IntegratorStateMustResolveToSignalObject=off  IntegratorRTWStateStorageClass=Auto  FilterContinuousStateAttributes=''  FilterStateMustResolveToSignalObject=off  FilterRTWStateStorageClass=Auto  ParallelPVariant=InternalParameters  IdealPVariant=Disabled  IVariant=InternalParameters  DVariant=Disabled  IntegratorVariant=Continuous  SatVariant=Disabled  AWVariant=Passthrough  PCopyVariant=Disabled  TRVariant=Disabled  FdbkBlocksVariant=Forward  IdealPFdbkVariant=Disabled  SatFdbkVariant=Disabled  DerivativeFilterVariant=Disabled  NVariant=Disabled  NCopyVariant=Disabled_SignalSpec  FilterICVariant=Disabled  IntegratorICVariant=InternalICs  ExternalResetVariant=Disabled  TRSumVariant=Passthrough  SumFdbkVariant=Disabled  SumVariant=Sum_PI  TsampFilterVariant=InternalTs  TsampNgainVariant=Passthrough  TsampIntegralVariant=Disabled_SignalSpec  ExternalSaturationOutDataTypeStr=Inherit: Same as second input
  PID Controller50 : slpidlib/PID Controller  Controller=PI  Form=Parallel  TimeDomain=Continuous-time  UseExternalTs=off  SampleTime=-1  IntegratorMethod=Forward Euler  FilterMethod=Forward Euler  ControllerParametersSource=internal  P=10  I=2000  UseKiTs=off  D=0  N=100  UseFilter=on  TunerSelectOption=Transfer Function Based (PID Tuner App)  InitialConditionSource=internal  InitialConditionForIntegrator=0  InitialConditionForFilter=0  DifferentiatorICPrevScaledInput=0  ExternalReset=none  TrackingMode=off  Kt=1  LimitOutput=off  SatLimitsSource=internal  UpperSaturationLimit=inf  LowerSaturationLimit=-inf  LinearizeAsGain=on  AntiWindupMode=none  Kb=1  LimitIntegrator=off  UpperIntegratorSaturationLimit=inf  LowerIntegratorSaturationLimit=-inf  POutMin=[]  POutMax=[]  IOutMin=[]  IOutMax=[]  DOutMin=[]  DOutMax=[]  NOutMin=[]  NOutMax=[]  SumOutMin=[]  SumOutMax=[]  SaturationOutMin=[]  SaturationOutMax=[]  PParamMin=[]  PParamMax=[]  IParamMin=[]  IParamMax=[]  DParamMin=[]  DParamMax=[]  NParamMin=[]  NParamMax=[]  KbParamMin=[]  KbParamMax=[]  KtParamMin=[]  KtParamMax=[]  KbOutMin=[]  KbOutMax=[]  KtOutMin=[]  KtOutMax=[]  IntegratorOutMin=[]  IntegratorOutMax=[]  FilterOutMin=[]  FilterOutMax=[]  SumI1OutMin=[]  SumI1OutMax=[]  SumI2OutMin=[]  SumI2OutMax=[]  SumI3OutMin=[]  SumI3OutMax=[]  SumI4OutMin=[]  SumI4OutMax=[]  SumDOutMin=[]  SumDOutMax=[]  DifferentiatorOutMin=[]  DifferentiatorOutMax=[]  FilterDiffOutCoefMin=[]  FilterDiffOutCoefMax=[]  ReciprocalOutMin=[]  ReciprocalOutMax=[]  SumDenOutMin=[]  SumDenOutMax=[]  SumNumOutMin=[]  SumNumOutMax=[]  DivideOutMin=[]  DivideOutMax=[]  UdiffTsProdOutMin=[]  UdiffTsProdOutMax=[]  NTsProdOutMin=[]  NTsProdOutMax=[]  UintegralTsProdOutMin=[]  UintegralTsProdOutMax=[]  UngainTsProdOutMin=[]  UngainTsProdOutMax=[]  ClampingZeroOutDataTypeStr=Inherit: Inherit via back propagation  ClampingZeroOutMin=[]  ClampingZeroOutMax=[]  FilterDenConstantOutDataTypeStr=Inherit: Inherit via back propagation  FilterDenConstantOutMin=[]  FilterDenConstantOutMax=[]  PCopyOutDataTypeStr=Inherit: Inherit via back propagation  PCopyOutMin=[]  PCopyOutMax=[]  NCopyOutDataTypeStr=Inherit: Inherit via back propagation  NCopyOutMin=[]  NCopyOutMax=[]  IntegratorContinuousStateAttributes=''  IntegratorStateMustResolveToSignalObject=off  IntegratorRTWStateStorageClass=Auto  FilterContinuousStateAttributes=''  FilterStateMustResolveToSignalObject=off  FilterRTWStateStorageClass=Auto  ParallelPVariant=InternalParameters  IdealPVariant=Disabled  IVariant=InternalParameters  DVariant=Disabled  IntegratorVariant=Continuous  SatVariant=Disabled  AWVariant=Passthrough  PCopyVariant=Disabled  TRVariant=Disabled  FdbkBlocksVariant=Forward  IdealPFdbkVariant=Disabled  SatFdbkVariant=Disabled  DerivativeFilterVariant=Disabled  NVariant=Disabled  NCopyVariant=Disabled_SignalSpec  FilterICVariant=Disabled  IntegratorICVariant=InternalICs  ExternalResetVariant=Disabled  TRSumVariant=Passthrough  SumFdbkVariant=Disabled  SumVariant=Sum_PI  TsampFilterVariant=InternalTs  TsampNgainVariant=Passthrough  TsampIntegralVariant=Disabled_SignalSpec  ExternalSaturationOutDataTypeStr=Inherit: Same as second input
  SVPWM Generator (2-Level)12 : spsSVPWMGenerator2LevelLib/SVPWM Generator (2-Level)  InputType=alpha-beta components  SwitchingPattern=Pattern #1  Fc=5000  ParUref=[0.8 -30 50]  Ts=0
  Scope56 : Scope  NumInputPorts=2
  Sum49 : Sum  Inputs=|+-
  Sum50 : Sum  Inputs=|+-
  Sum51 : Sum  Inputs=|+-
  Terminator22 : Terminator
  Terminator23 : Terminator
  abc to Alpha-Beta-Zero11 : spsabctoAlphaBetaZeroLib/abc to Alpha-Beta-Zero
  dq0 to Alpha-Beta-Zero11 : spsdq0toAlphaBetaZeroLib/dq0 to Alpha-Beta-Zero  Alignment=90 degrees behind phase A axis
  Gates : Outport
  wires:
  <Rotor angle thetam (rad)>/1 -> Gain34/1
  Mux23/1 -> dq0 to Alpha-Beta-Zero11/1
  Demux24/3 -> Terminator23/1
  Alpha-Beta-Zero to dq11/1 -> Demux24/1
  Constant55/1 -> Mux23/3
  Demux24/2 -> Sum50/2
  Mux24/1 -> abc to Alpha-Beta-Zero11/1
  <Rotor speed wm (rad/s)>/1 -> Gain35/1
  Constant52/1 -> Sum49/1
  Sum51/1 -> PID Controller48/1
  Gain34/1 -> Alpha-Beta-Zero to dq11/2, dq0 to Alpha-Beta-Zero11/2
  Gain35/1 -> Sum51/2
  PID Controller49/1 -> Mux23/1
  SVPWM Generator (2-Level)12/1 -> Gates/1
  abc to Alpha-Beta-Zero11/1 -> Alpha-Beta-Zero to dq11/1
  <Stator current is_a (A)>/1 -> Mux24/1
  <Stator current is_c (A)>/1 -> Mux24/3
  PID Controller50/1 -> Mux23/2
  dq0 to Alpha-Beta-Zero11/1 -> Demux23/1
  <Stator current is_b (A)>/1 -> Mux24/2
  Demux23/1 -> SVPWM Generator (2-Level)12/1
  Sum49/1 -> Scope56/2, PID Controller49/1
  Demux24/1 -> Sum49/2
  Demux23/2 -> SVPWM Generator (2-Level)12/2
  Speed_Ref/1 -> Sum51/1
  Demux23/3 -> Terminator22/1
  Sum50/1 -> PID Controller50/1
  PID Controller48/1 -> Scope56/1, Sum50/1

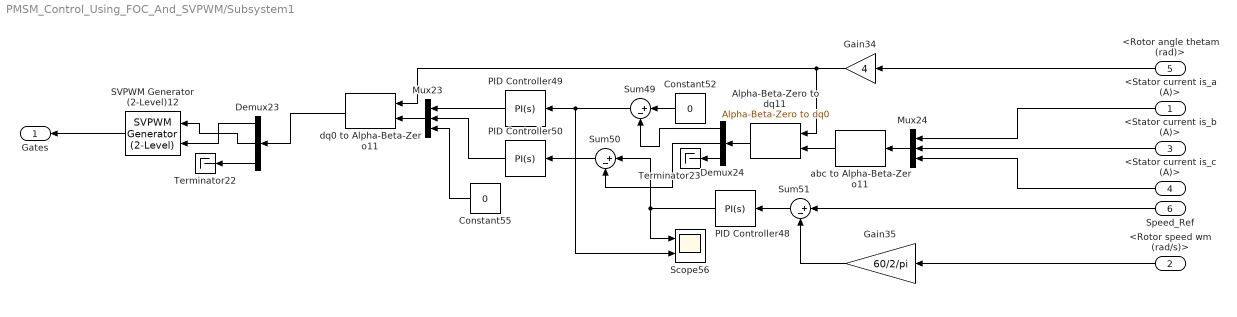
== system PMSM_Control_Using_FOC_And_SVPWM/Subsystem1 ==
  <Stator current is_a (A)> : Inport
  <Rotor speed wm (rad/s)> : Inport  Port=2
  <Stator current is_b (A)> : Inport  Port=3
  <Stator current is_c (A)> : Inport  Port=4
  <Rotor angle thetam (rad)> : Inport  Port=5
  Speed_Ref : Inport  Port=6
  Alpha-Beta-Zero to dq11 : spsAlphaBetaZerotodq0Lib/Alpha-Beta-Zero to dq0  Alignment=90 degrees behind phase A axis
  Constant52 : Constant  Value=0
  Constant55 : Constant  Value=0
  Demux23 : Demux  Outputs=3
  Demux24 : Demux  Outputs=3
  Gain34 : Gain  Gain=4
  Gain35 : Gain  Gain=60/2/pi
  Mux23 : Mux  Inputs=3
  Mux24 : Mux  Inputs=3
  PID Controller48 : slpidlib/PID Controller  Controller=PI  Form=Parallel  TimeDomain=Continuous-time  UseExternalTs=off  SampleTime=-1  IntegratorMethod=Forward Euler  FilterMethod=Forward Euler  ControllerParametersSource=internal  P=0.5  I=10  UseKiTs=off  D=0  N=100  UseFilter=on  TunerSelectOption=Transfer Function Based (PID Tuner App)  InitialConditionSource=internal  InitialConditionForIntegrator=0  InitialConditionForFilter=0  DifferentiatorICPrevScaledInput=0  ExternalReset=none  TrackingMode=off  Kt=1  LimitOutput=off  SatLimitsSource=internal  UpperSaturationLimit=inf  LowerSaturationLimit=-inf  LinearizeAsGain=on  AntiWindupMode=none  Kb=1  LimitIntegrator=off  UpperIntegratorSaturationLimit=inf  LowerIntegratorSaturationLimit=-inf  POutMin=[]  POutMax=[]  IOutMin=[]  IOutMax=[]  DOutMin=[]  DOutMax=[]  NOutMin=[]  NOutMax=[]  SumOutMin=[]  SumOutMax=[]  SaturationOutMin=[]  SaturationOutMax=[]  PParamMin=[]  PParamMax=[]  IParamMin=[]  IParamMax=[]  DParamMin=[]  DParamMax=[]  NParamMin=[]  NParamMax=[]  KbParamMin=[]  KbParamMax=[]  KtParamMin=[]  KtParamMax=[]  KbOutMin=[]  KbOutMax=[]  KtOutMin=[]  KtOutMax=[]  IntegratorOutMin=[]  IntegratorOutMax=[]  FilterOutMin=[]  FilterOutMax=[]  SumI1OutMin=[]  SumI1OutMax=[]  SumI2OutMin=[]  SumI2OutMax=[]  SumI3OutMin=[]  SumI3OutMax=[]  SumI4OutMin=[]  SumI4OutMax=[]  SumDOutMin=[]  SumDOutMax=[]  DifferentiatorOutMin=[]  DifferentiatorOutMax=[]  FilterDiffOutCoefMin=[]  FilterDiffOutCoefMax=[]  ReciprocalOutMin=[]  ReciprocalOutMax=[]  SumDenOutMin=[]  SumDenOutMax=[]  SumNumOutMin=[]  SumNumOutMax=[]  DivideOutMin=[]  DivideOutMax=[]  UdiffTsProdOutMin=[]  UdiffTsProdOutMax=[]  NTsProdOutMin=[]  NTsProdOutMax=[]  UintegralTsProdOutMin=[]  UintegralTsProdOutMax=[]  UngainTsProdOutMin=[]  UngainTsProdOutMax=[]  ClampingZeroOutDataTypeStr=Inherit: Inherit via back propagation  ClampingZeroOutMin=[]  ClampingZeroOutMax=[]  FilterDenConstantOutDataTypeStr=Inherit: Inherit via back propagation  FilterDenConstantOutMin=[]  FilterDenConstantOutMax=[]  PCopyOutDataTypeStr=Inherit: Inherit via back propagation  PCopyOutMin=[]  PCopyOutMax=[]  NCopyOutDataTypeStr=Inherit: Inherit via back propagation  NCopyOutMin=[]  NCopyOutMax=[]  IntegratorContinuousStateAttributes=''  IntegratorStateMustResolveToSignalObject=off  IntegratorRTWStateStorageClass=Auto  FilterContinuousStateAttributes=''  FilterStateMustResolveToSignalObject=off  FilterRTWStateStorageClass=Auto  ParallelPVariant=InternalParameters  IdealPVariant=Disabled  IVariant=InternalParameters  DVariant=Disabled  IntegratorVariant=Continuous  SatVariant=Disabled  AWVariant=Passthrough  PCopyVariant=Disabled  TRVariant=Disabled  FdbkBlocksVariant=Forward  IdealPFdbkVariant=Disabled  SatFdbkVariant=Disabled  DerivativeFilterVariant=Disabled  NVariant=Disabled  NCopyVariant=Disabled_SignalSpec  FilterICVariant=Disabled  IntegratorICVariant=InternalICs  ExternalResetVariant=Disabled  TRSumVariant=Passthrough  SumFdbkVariant=Disabled  SumVariant=Sum_PI  TsampFilterVariant=InternalTs  TsampNgainVariant=Passthrough  TsampIntegralVariant=Disabled_SignalSpec  ExternalSaturationOutDataTypeStr=Inherit: Same as second input
  PID Controller49 : slpidlib/PID Controller  Controller=PI  Form=Parallel  TimeDomain=Continuous-time  UseExternalTs=off  SampleTime=-1  IntegratorMethod=Forward Euler  FilterMethod=Forward Euler  ControllerParametersSource=internal  P=10  I=2000  UseKiTs=off  D=0  N=100  UseFilter=on  TunerSelectOption=Transfer Function Based (PID Tuner App)  InitialConditionSource=internal  InitialConditionForIntegrator=0  InitialConditionForFilter=0  DifferentiatorICPrevScaledInput=0  ExternalReset=none  TrackingMode=off  Kt=1  LimitOutput=off  SatLimitsSource=internal  UpperSaturationLimit=inf  LowerSaturationLimit=-inf  LinearizeAsGain=on  AntiWindupMode=none  Kb=1  LimitIntegrator=off  UpperIntegratorSaturationLimit=inf  LowerIntegratorSaturationLimit=-inf  POutMin=[]  POutMax=[]  IOutMin=[]  IOutMax=[]  DOutMin=[]  DOutMax=[]  NOutMin=[]  NOutMax=[]  SumOutMin=[]  SumOutMax=[]  SaturationOutMin=[]  SaturationOutMax=[]  PParamMin=[]  PParamMax=[]  IParamMin=[]  IParamMax=[]  DParamMin=[]  DParamMax=[]  NParamMin=[]  NParamMax=[]  KbParamMin=[]  KbParamMax=[]  KtParamMin=[]  KtParamMax=[]  KbOutMin=[]  KbOutMax=[]  KtOutMin=[]  KtOutMax=[]  IntegratorOutMin=[]  IntegratorOutMax=[]  FilterOutMin=[]  FilterOutMax=[]  SumI1OutMin=[]  SumI1OutMax=[]  SumI2OutMin=[]  SumI2OutMax=[]  SumI3OutMin=[]  SumI3OutMax=[]  SumI4OutMin=[]  SumI4OutMax=[]  SumDOutMin=[]  SumDOutMax=[]  DifferentiatorOutMin=[]  DifferentiatorOutMax=[]  FilterDiffOutCoefMin=[]  FilterDiffOutCoefMax=[]  ReciprocalOutMin=[]  ReciprocalOutMax=[]  SumDenOutMin=[]  SumDenOutMax=[]  SumNumOutMin=[]  SumNumOutMax=[]  DivideOutMin=[]  DivideOutMax=[]  UdiffTsProdOutMin=[]  UdiffTsProdOutMax=[]  NTsProdOutMin=[]  NTsProdOutMax=[]  UintegralTsProdOutMin=[]  UintegralTsProdOutMax=[]  UngainTsProdOutMin=[]  UngainTsProdOutMax=[]  ClampingZeroOutDataTypeStr=Inherit: Inherit via back propagation  ClampingZeroOutMin=[]  ClampingZeroOutMax=[]  FilterDenConstantOutDataTypeStr=Inherit: Inherit via back propagation  FilterDenConstantOutMin=[]  FilterDenConstantOutMax=[]  PCopyOutDataTypeStr=Inherit: Inherit via back propagation  PCopyOutMin=[]  PCopyOutMax=[]  NCopyOutDataTypeStr=Inherit: Inherit via back propagation  NCopyOutMin=[]  NCopyOutMax=[]  IntegratorContinuousStateAttributes=''  IntegratorStateMustResolveToSignalObject=off  IntegratorRTWStateStorageClass=Auto  FilterContinuousStateAttributes=''  FilterStateMustResolveToSignalObject=off  FilterRTWStateStorageClass=Auto  ParallelPVariant=InternalParameters  IdealPVariant=Disabled  IVariant=InternalParameters  DVariant=Disabled  IntegratorVariant=Continuous  SatVariant=Disabled  AWVariant=Passthrough  PCopyVariant=Disabled  TRVariant=Disabled  FdbkBlocksVariant=Forward  IdealPFdbkVariant=Disabled  SatFdbkVariant=Disabled  DerivativeFilterVariant=Disabled  NVariant=Disabled  NCopyVariant=Disabled_SignalSpec  FilterICVariant=Disabled  IntegratorICVariant=InternalICs  ExternalResetVariant=Disabled  TRSumVariant=Passthrough  SumFdbkVariant=Disabled  SumVariant=Sum_PI  TsampFilterVariant=InternalTs  TsampNgainVariant=Passthrough  TsampIntegralVariant=Disabled_SignalSpec  ExternalSaturationOutDataTypeStr=Inherit: Same as second input
  PID Controller50 : slpidlib/PID Controller  Controller=PI  Form=Parallel  TimeDomain=Continuous-time  UseExternalTs=off  SampleTime=-1  IntegratorMethod=Forward Euler  FilterMethod=Forward Euler  ControllerParametersSource=internal  P=10  I=2000  UseKiTs=off  D=0  N=100  UseFilter=on  TunerSelectOption=Transfer Function Based (PID Tuner App)  InitialConditionSource=internal  InitialConditionForIntegrator=0  InitialConditionForFilter=0  DifferentiatorICPrevScaledInput=0  ExternalReset=none  TrackingMode=off  Kt=1  LimitOutput=off  SatLimitsSource=internal  UpperSaturationLimit=inf  LowerSaturationLimit=-inf  LinearizeAsGain=on  AntiWindupMode=none  Kb=1  LimitIntegrator=off  UpperIntegratorSaturationLimit=inf  LowerIntegratorSaturationLimit=-inf  POutMin=[]  POutMax=[]  IOutMin=[]  IOutMax=[]  DOutMin=[]  DOutMax=[]  NOutMin=[]  NOutMax=[]  SumOutMin=[]  SumOutMax=[]  SaturationOutMin=[]  SaturationOutMax=[]  PParamMin=[]  PParamMax=[]  IParamMin=[]  IParamMax=[]  DParamMin=[]  DParamMax=[]  NParamMin=[]  NParamMax=[]  KbParamMin=[]  KbParamMax=[]  KtParamMin=[]  KtParamMax=[]  KbOutMin=[]  KbOutMax=[]  KtOutMin=[]  KtOutMax=[]  IntegratorOutMin=[]  IntegratorOutMax=[]  FilterOutMin=[]  FilterOutMax=[]  SumI1OutMin=[]  SumI1OutMax=[]  SumI2OutMin=[]  SumI2OutMax=[]  SumI3OutMin=[]  SumI3OutMax=[]  SumI4OutMin=[]  SumI4OutMax=[]  SumDOutMin=[]  SumDOutMax=[]  DifferentiatorOutMin=[]  DifferentiatorOutMax=[]  FilterDiffOutCoefMin=[]  FilterDiffOutCoefMax=[]  ReciprocalOutMin=[]  ReciprocalOutMax=[]  SumDenOutMin=[]  SumDenOutMax=[]  SumNumOutMin=[]  SumNumOutMax=[]  DivideOutMin=[]  DivideOutMax=[]  UdiffTsProdOutMin=[]  UdiffTsProdOutMax=[]  NTsProdOutMin=[]  NTsProdOutMax=[]  UintegralTsProdOutMin=[]  UintegralTsProdOutMax=[]  UngainTsProdOutMin=[]  UngainTsProdOutMax=[]  ClampingZeroOutDataTypeStr=Inherit: Inherit via back propagation  ClampingZeroOutMin=[]  ClampingZeroOutMax=[]  FilterDenConstantOutDataTypeStr=Inherit: Inherit via back propagation  FilterDenConstantOutMin=[]  FilterDenConstantOutMax=[]  PCopyOutDataTypeStr=Inherit: Inherit via back propagation  PCopyOutMin=[]  PCopyOutMax=[]  NCopyOutDataTypeStr=Inherit: Inherit via back propagation  NCopyOutMin=[]  NCopyOutMax=[]  IntegratorContinuousStateAttributes=''  IntegratorStateMustResolveToSignalObject=off  IntegratorRTWStateStorageClass=Auto  FilterContinuousStateAttributes=''  FilterStateMustResolveToSignalObject=off  FilterRTWStateStorageClass=Auto  ParallelPVariant=InternalParameters  IdealPVariant=Disabled  IVariant=InternalParameters  DVariant=Disabled  IntegratorVariant=Continuous  SatVariant=Disabled  AWVariant=Passthrough  PCopyVariant=Disabled  TRVariant=Disabled  FdbkBlocksVariant=Forward  IdealPFdbkVariant=Disabled  SatFdbkVariant=Disabled  DerivativeFilterVariant=Disabled  NVariant=Disabled  NCopyVariant=Disabled_SignalSpec  FilterICVariant=Disabled  IntegratorICVariant=InternalICs  ExternalResetVariant=Disabled  TRSumVariant=Passthrough  SumFdbkVariant=Disabled  SumVariant=Sum_PI  TsampFilterVariant=InternalTs  TsampNgainVariant=Passthrough  TsampIntegralVariant=Disabled_SignalSpec  ExternalSaturationOutDataTypeStr=Inherit: Same as second input
  SVPWM Generator (2-Level)12 : spsSVPWMGenerator2LevelLib/SVPWM Generator (2-Level)  InputType=alpha-beta components  SwitchingPattern=Pattern #1  Fc=5000  ParUref=[0.8 -30 50]  Ts=0
  Scope56 : Scope  NumInputPorts=2
  Sum49 : Sum  Inputs=|+-
  Sum50 : Sum  Inputs=|+-
  Sum51 : Sum  Inputs=|+-
  Terminator22 : Terminator
  Terminator23 : Terminator
  abc to Alpha-Beta-Zero11 : spsabctoAlphaBetaZeroLib/abc to Alpha-Beta-Zero
  dq0 to Alpha-Beta-Zero11 : spsdq0toAlphaBetaZeroLib/dq0 to Alpha-Beta-Zero  Alignment=90 degrees behind phase A axis
  Gates : Outport
  wires:
  <Rotor angle thetam (rad)>/1 -> Gain34/1
  Mux23/1 -> dq0 to Alpha-Beta-Zero11/1
  Demux24/3 -> Terminator23/1
  Alpha-Beta-Zero to dq11/1 -> Demux24/1
  Constant55/1 -> Mux23/3
  Demux24/2 -> Sum50/2
  Mux24/1 -> abc to Alpha-Beta-Zero11/1
  <Rotor speed wm (rad/s)>/1 -> Gain35/1
  Constant52/1 -> Sum49/1
  Sum51/1 -> PID Controller48/1
  Gain34/1 -> Alpha-Beta-Zero to dq11/2, dq0 to Alpha-Beta-Zero11/2
  Gain35/1 -> Sum51/2
  PID Controller49/1 -> Mux23/1
  SVPWM Generator (2-Level)12/1 -> Gates/1
  abc to Alpha-Beta-Zero11/1 -> Alpha-Beta-Zero to dq11/1
  <Stator current is_a (A)>/1 -> Mux24/1
  <Stator current is_c (A)>/1 -> Mux24/3
  PID Controller50/1 -> Mux23/2
  dq0 to Alpha-Beta-Zero11/1 -> Demux23/1
  <Stator current is_b (A)>/1 -> Mux24/2
  Demux23/1 -> SVPWM Generator (2-Level)12/1
  Sum49/1 -> Scope56/2, PID Controller49/1
  Demux24/1 -> Sum49/2
  Demux23/2 -> SVPWM Generator (2-Level)12/2
  Speed_Ref/1 -> Sum51/1
  Demux23/3 -> Terminator22/1
  Sum50/1 -> PID Controller50/1
  PID Controller48/1 -> Scope56/1, Sum50/1

== system PMSM_Control_Using_FOC_And_SVPWM/Torque_Input ==
  Demux : Demux  Tag=STV Demux  Outputs=1
      settings: DisplayOption=none
  FromWs : FromWorkspace  Tag=STV FromWs  VariableName=tuvar
      SigBuilderData=|
      | common.afterFinalStr = 'Extrapolate'
      | common.sampleTime = 0
      | dataSet.timeRange = [0 2.5]
      | dataSet.name = 'Flat_Road_Torque'
      | sbobj.Name = 'Signal Builder'
      | sbobj.Groups.Name = 'Flat_Road_Torque'
      | sbobj.Groups.Signals.Name = 'torque'
      | sbobj.Groups.Signals.XData = [0 0.05 0.1 0.3 0.4 0.7 0.8 1.2 1.25 1.6 1.65 2 2.05 2.25 2.35 2.5]
      | sbobj.Groups.Signals.YData = [0 0 5 5 3 3 -5 -5 -3 -3 -4 -4 -5 -5 -1 -1]
      | sbobj.Groups.TimeRange = [0 2.5]
  torque : Outport  VectorParamsAs1DForOutWhenUnconnected=off
  wires:
  FromWs/1 -> Demux/1
  Demux/1 -> torque/1

== system PMSM_Control_Using_FOC_And_SVPWM/Torque_Input1 ==
  Demux : Demux  Tag=STV Demux  Outputs=1
      settings: DisplayOption=none
  FromWs : FromWorkspace  Tag=STV FromWs  VariableName=tuvar
      SigBuilderData=|
      | common.afterFinalStr = 'Extrapolate'
      | common.sampleTime = 0
      | dataSet.timeRange = [0 2.5]
      | dataSet.name = 'Flat_Road_Torque'
      | sbobj.Name = 'Signal Builder'
      | sbobj.Groups.Name = 'Flat_Road_Torque'
      | sbobj.Groups.Signals.Name = 'torque'
      | sbobj.Groups.Signals.XData = [0 0.05 0.1 0.3 0.4 0.7 0.8 1.2 1.25 1.6 1.65 2 2.05 2.25 2.35 2.5]
      | sbobj.Groups.Signals.YData = [0 0 5 5 3 3 -5 -5 -3 -3 -4 -4 -5 -5 -1 -1]
      | sbobj.Groups.TimeRange = [0 2.5]
  torque : Outport  VectorParamsAs1DForOutWhenUnconnected=off
  wires:
  FromWs/1 -> Demux/1
  Demux/1 -> torque/1
